simulink model "CheckBrakeDistance"  (R2014a)
settings: Solver=ode3  SolverMode=SingleTasking  StartTime=0.0  StopTime=inf  RelTol=1e-3
libraries: canoelib x4, simulink x2
settings Model: targetArch=x86  analysisModel=0  XcpMessageLength=-1  hasCAPLCallBlock=0  Creator=visjf  LastModifiedBy=vikafla
settings DataIOCC: SignalLoggingSaveFormat=ModelDataLogs
settings OptimizationCC: ExpressionDepthLimit=2147483647  InitFltsAndDblsToZero=on
settings DebuggingCC: UnderspecifiedInitializationDetection=Classic  MultiTaskCondExecSysMsg=none  FcnCallInpInsideContextMsg=UseLocalSettings  StateNameClashWarn=warning
settings HardwareCC: TargetHWDeviceType=32-bit Generic
settings RTWCC: SystemTargetFile=cn.tlc  TemplateMakefile=cn_msdll.tmf  Description=Vector CANoe Real-Time Target DLL (Visual C/C++ Project Makefile)  ProcessScript=cn_make_rtw_hook  IncludeERTFirstTime=on
settings STFCustomTargetCC: TargetFcnLib=ansi_tfl_tmw.mat  ModelReferenceCompliant=off  ConcurrentExecutionCompliant=off  MatFileLogging=on  CPPClassGenCompliant=on  SystemTargetFile=cn.tlc
settings GRTTargetCC: TargetFcnLib=ansi_tfl_tmw.mat  ModelReferenceCompliant=off  ParMdlRefBuildCompliant=off  CompOptLevelCompliant=off  ConcurrentExecutionCompliant=off  CombineOutputUpdateFcns=off  GRTInterface=on  ExtModeMexFile=noextcomm  RTWCAPISignals=on  RTWCAPIParams=on

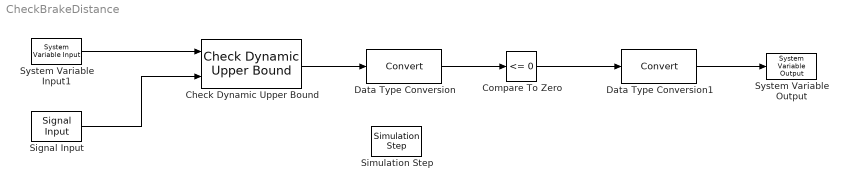
== system CheckBrakeDistance ==
  Check Dynamic Upper Bound : simulink/Model Verification/Check Dynamic  Upper Bound  Description=sig < max  enabled=on  stopWhenAssertionFail=off  export=on  icon=graphic
  Compare To Zero : simulink/Logic and Bit Operations/Compare To Zero  relop=<=  OutDataTypeStr=uint8  ZeroCross=off
  Data Type Conversion : DataTypeConversion
  Data Type Conversion1 : DataTypeConversion
  Signal Input : canoelib/CANoe I//O/Signal Input  dbName=""  nodeName=""  msgName=""  sigName=xF  editSampleTime=0  rawValue=Physical value  dataType=Default  dataTypeDB=unknown  hasEncoding=off
      settings: AttributesFormatString=%<sigName>
  Simulation Step : canoelib/CANoe I//O/Simulation Step  mode=Synchronized
      settings: AttributesFormatString=%<mode>
  System Variable Input1 : canoelib/CANoe I//O/System Variable Input  nsName=MatlabIO  sysVarName=SetPointBrakeDist  arrayIndex=-1  editSampleTime=0  rawValue=Default  dataType=Default  dataTypeDB=unknown  hasEncoding=off  dataTypeCANoe=Get from CANoe
      settings: AttributesFormatString=%<nsName>::%<sysVarName>
  System Variable Output : canoelib/CANoe I//O/System Variable Output  nsName=MatlabIO  sysVarName=BrakeDistVerdict  arrayIndex=-1  rawValue=Default  dataType=Default  dataTypeDB=unknown  hasEncoding=off  dataTypeCANoe=Get from CANoe
      settings: AttributesFormatString=%<nsName>::%<sysVarName>
  wires:
  System Variable Input1/1 -> Check Dynamic Upper Bound/1
  Signal Input/1 -> Check Dynamic Upper Bound/2
  Check Dynamic Upper Bound/1 -> Data Type Conversion/1
  Data Type Conversion/1 -> Compare To Zero/1
  Compare To Zero/1 -> Data Type Conversion1/1
  Data Type Conversion1/1 -> System Variable Output/1
